simulink model "bdot_simple_sim_edits"  (R2016b)
settings: Solver=ode23tb  StartTime=0.0  StopTime=2000  RelTol=1e-3  EnableMultiTasking=on
values from neighbouring files (symbols this model uses):
  fsw_params = init_fsw_params()    [bdot_controller_edit_test.m]    (also in bdot_controlller_unit_test.m)
  sim_params = init_sim_params(fsw_params)    [bdot_controller_edit_test.m]    (also in bdot_controlller_unit_test.m)
undefined symbols (not defined in the file or in its folder): body_rates, DiscIntNeverNeededParam, Dynamics, dynamics_lib, position, quaternion, velocity
libraries: aerolibutil x11, vrlib x2, bus_stubs_template x1, environment_lib x1, bdot_controller_lib x1, magnetorquer_assembly_lib x1
settings Model: Creator=Taylor  LastModifiedBy=taylorreynolds
settings OptimizationCC: DefaultParameterBehavior=Inlined  UseDivisionForNetSlopeComputation=on  UseFloatMulNetSlope=on  InlineInvariantSignals=on  PassReuseOutputArgsAs=Individual arguments  ZeroExternalMemoryAtStartup=off  ZeroInternalMemoryAtStartup=off  NoFixptDivByZeroProtection=on  EfficientFloat2IntCast=on  LifeSpan=1
settings DebuggingCC: ParameterTunabilityLossMsg=error  SFUnexpectedBacktrackingDiag=warning  SFNoUnconditionalDefaultTransitionDiag=warning  SFExecutionAtInitializationDiag=none
settings HardwareCC: ProdBitPerInt=16  ProdBitPerPointer=16  ProdBitPerSizeT=16  ProdBitPerPtrDiffT=16  ProdLargestAtomicFloat=None  ProdWordSize=16  ProdHWDeviceType=Texas Instruments->MSP430
settings RTWCC: SystemTargetFile=ert.tlc  TemplateMakefile=ert_default_tmf  Description=Embedded Coder  GenerateReport=on  IncludeHyperlinkInReport=on  LaunchReport=on  GenerateTraceInfo=on  GenerateTraceReport=on  GenerateTraceReportSl=on  GenerateTraceReportSf=on  GenerateTraceReportEml=on  GenerateCodeMetricsReport=on
settings CodeAppCC: ForceParamTrailComments=on  IgnoreCustomStorageClasses=off  OperatorAnnotations=on  SimulinkDataObjDesc=on  SFDataObjDesc=on  MATLABFcnDesc=on  CustomSymbolStrGlobalVar=rt$N$M  CustomSymbolStrType=$N$M  CustomSymbolStrFcn=$N$M$F  CustomSymbolStrMacro=$N$M  InsertBlockDesc=on  MATLABSourceComments=on
settings ERTTargetCC: GenerateSampleERTMain=on  CombineSignalStateStructs=on  SupportComplex=off  SupportContinuousTime=on  SupportNonInlinedSFcns=on  InlinedParameterPlacement=NonHierarchical  ERTCustomFileTemplate=example_file_process.tlc  ERTFilePackagingFormat=CompactWithDataFile
settings ConfigComp: CovMetricSettings=dw  CovHtmlReporting=on  CovSaveCumulativeToWorkspaceVar=on  CovSaveSingleToWorkspaceVar=on  CovExternalEMLEnable=off

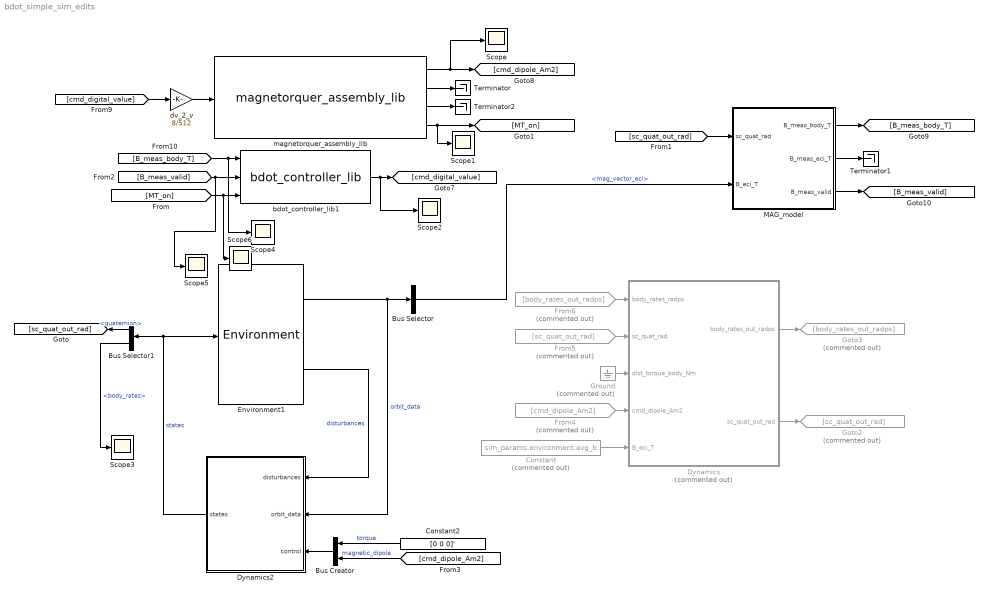
== system bdot_simple_sim_edits ==
  Bus Creator : BusCreator  Inputs=2
  Bus Selector : BusSelector  OutputSignals=mag_vector_eci
  Bus Selector1 : BusSelector  OutputSignals=quaternion,body_rates
  Constant : Constant  Commented=on  Value=sim_params.environment.avg_b
  Constant2 : Constant  Value=[0 0 0]'
  Dynamics : Subsystem  Commented=on
  Dynamics2 : Subsystem  AncestorBlock=dynamics_lib/Dynamics
  Environment1 : environment_lib/Environment
  From4 : From  Commented=on  GotoTag=cmd_dipole_Am2
  From5 : From  Commented=on  GotoTag=sc_quat_out_rad
  From6 : From  Commented=on  GotoTag=body_rates_out_radps
  Goto2 : Goto  Commented=on  GotoTag=sc_quat_out_rad
  Goto3 : Goto  Commented=on  GotoTag=body_rates_out_radps
  Ground : Ground  Commented=on
  MAG_model : Subsystem
  Scope{,1..6} (7 alike) : Scope
  Terminator : Terminator
  Terminator1 : Terminator
  Terminator2 : Terminator
  bdot_controller_lib1 : bdot_controller_lib/bdot_controller_lib
  dv_2_v : Gain  Gain=8/512
  magnetorquer_assembly_lib : magnetorquer_assembly_lib/magnetorquer_assembly_lib
  wires:
  bdot_controller_lib1/1 -> Scope2/1, [cmd_digital_value]
  [B_meas_body_T] -> Scope4/1, bdot_controller_lib1/1
  MAG_model/3(B_meas_valid) -> [B_meas_valid]
  MAG_model/1(B_meas_body_T) -> [B_meas_body_T]
  MAG_model/2(B_meas_eci_T) -> Terminator1/1
  [sc_quat_out_rad] -> MAG_model/1(sc_quat_rad)
  From6/1 -> Dynamics/1(body_rates_radps)
  Dynamics/1(body_rates_out_radps) -> Goto3/1
  Dynamics/2(sc_quat_out_rad) -> Goto2/1
  From5/1 -> Dynamics/2(sc_quat_rad)
  Ground/1 -> Dynamics/3(dist_torque_body_Nm)
  From4/1 -> Dynamics/4(cmd_dipole_Am2)
  Constant/1 -> Dynamics/5(B_eci_T)
  [B_meas_valid] -> Scope5/1, bdot_controller_lib1/2
  dv_2_v/1 -> magnetorquer_assembly_lib/1
  [cmd_digital_value] -> dv_2_v/1
  magnetorquer_assembly_lib/1 -> Scope/1, [cmd_dipole_Am2]
  magnetorquer_assembly_lib/2 -> Terminator/1
  magnetorquer_assembly_lib/4 -> Scope1/1, [MT_on]
  magnetorquer_assembly_lib/3 -> Terminator2/1
  [MT_on] -> Scope6/1, bdot_controller_lib1/3
  Environment1/1 -> Dynamics2/2(orbit_data), Bus Selector/1  "orbit_data"
  Environment1/2 -> Dynamics2/1(disturbances)  "disturbances"
  Bus Creator/1 -> Dynamics2/3(control)
  Dynamics2/1(states) -> Environment1/1, Bus Selector1/1  "states"
  Constant2/1 -> Bus Creator/1  "torque"
  [cmd_dipole_Am2] -> Bus Creator/2  "magnetic_dipole"
  Bus Selector/1 -> MAG_model/2(B_eci_T)  "<mag_vector_eci>"
  Bus Selector1/1 -> [sc_quat_out_rad]  "<quaternion>"
  Bus Selector1/2 -> Scope3/1  "<body_rates>"

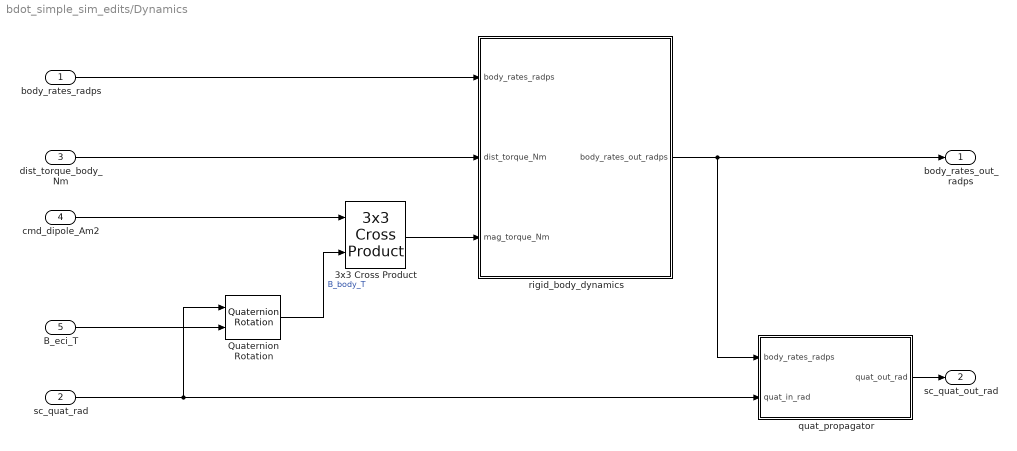
== system bdot_simple_sim_edits/Dynamics ==
  body_rates_radps : Inport
  sc_quat_rad : Inport  Port=2
  dist_torque_body_Nm : Inport  Port=3
  cmd_dipole_Am2 : Inport  Port=4
  B_eci_T : Inport  Port=5
  3x3 Cross Product : aerolibutil/3x3 Cross Product
  Quaternion Rotation : aerolibutil/Quaternion Rotation
  quat_propagator : Subsystem
  rigid_body_dynamics : Subsystem
  body_rates_out_radps : Outport
  sc_quat_out_rad : Outport  Port=2
  wires:
  Quaternion Rotation/1 -> 3x3 Cross Product/2  "B_body_T"
  cmd_dipole_Am2/1 -> 3x3 Cross Product/1
  dist_torque_body_Nm/1 -> rigid_body_dynamics/2(dist_torque_Nm)
  sc_quat_rad/1 -> Quaternion Rotation/1, quat_propagator/2(quat_in_rad)
  quat_propagator/1(quat_out_rad) -> sc_quat_out_rad/1
  body_rates_radps/1 -> rigid_body_dynamics/1(body_rates_radps)
  rigid_body_dynamics/1(body_rates_out_radps) -> body_rates_out_radps/1, quat_propagator/1(body_rates_radps)
  B_eci_T/1 -> Quaternion Rotation/2
  3x3 Cross Product/1 -> rigid_body_dynamics/3(mag_torque_Nm)

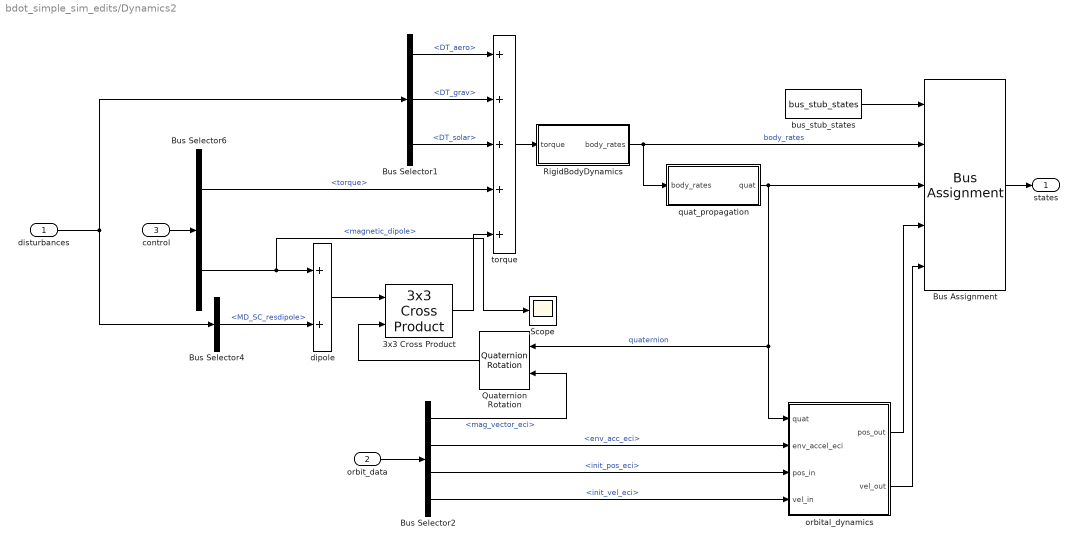
== system bdot_simple_sim_edits/Dynamics2 ==
  disturbances : Inport  OutDataTypeStr=Bus: disturbances
  orbit_data : Inport  Port=2  OutDataTypeStr=Bus: orbit_data
  control : Inport  Port=3  OutDataTypeStr=Bus: control
  3x3 Cross Product : aerolibutil/3x3 Cross Product
  Bus Assignment : BusAssignment  AssignedSignals=body_rates,quaternion,position,velocity
  Bus Selector1 : BusSelector  OutputSignals=DT_aero,DT_grav,DT_solar
  Bus Selector2 : BusSelector  OutputSignals=mag_vector_eci,env_acc_eci,init_pos_eci,init_vel_eci
  Bus Selector4 : BusSelector  OutputSignals=MD_SC_resdipole
  Bus Selector6 : BusSelector  OutputSignals=torque,magnetic_dipole
  Quaternion Rotation : aerolibutil/Quaternion Rotation
  RigidBodyDynamics : Subsystem
  Scope : Scope
  bus_stub_states : bus_stubs_template/bus_stub_states
  dipole : Sum  Inputs=2
  orbital_dynamics : Subsystem
  quat_propagation : Subsystem
  torque : Sum  Inputs=5
  states : Outport
  wires:
  orbit_data/1 -> Bus Selector2/1
  Bus Selector2/4 -> orbital_dynamics/4(vel_in)  "<init_vel_eci>"
  Bus Selector2/3 -> orbital_dynamics/3(pos_in)  "<init_pos_eci>"
  orbital_dynamics/1(pos_out) -> Bus Assignment/4
  orbital_dynamics/2(vel_out) -> Bus Assignment/5
  Bus Selector2/1 -> Quaternion Rotation/2  "<mag_vector_eci>"
  Bus Selector2/2 -> orbital_dynamics/2(env_accel_eci)  "<env_acc_eci>"
  3x3 Cross Product/1 -> torque/5
  Quaternion Rotation/1 -> 3x3 Cross Product/2
  dipole/1 -> 3x3 Cross Product/1
  torque/1 -> RigidBodyDynamics/1(torque)
  Bus Selector6/2 -> Scope/1, dipole/1  "<magnetic_dipole>"
  Bus Selector4/1 -> dipole/2  "<MD_SC_resdipole>"
  Bus Selector6/1 -> torque/4  "<torque>"
  control/1 -> Bus Selector6/1
  Bus Selector1/3 -> torque/3  "<DT_solar>"
  Bus Selector1/2 -> torque/2  "<DT_grav>"
  Bus Selector1/1 -> torque/1  "<DT_aero>"
  disturbances/1 -> Bus Selector1/1, Bus Selector4/1
  RigidBodyDynamics/1(body_rates) -> quat_propagation/1(body_rates), Bus Assignment/2  "body_rates"
  quat_propagation/1(quat) -> orbital_dynamics/1(quat), Quaternion Rotation/1, Bus Assignment/3  "quaternion"
  bus_stub_states/1 -> Bus Assignment/1
  Bus Assignment/1 -> states/1

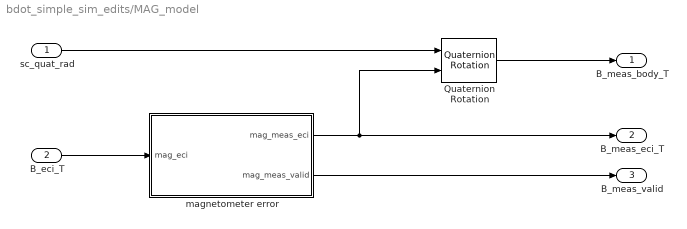
== system bdot_simple_sim_edits/MAG_model ==
  sc_quat_rad : Inport
  B_eci_T : Inport  Port=2
  Quaternion Rotation : aerolibutil/Quaternion Rotation
  magnetometer error : Subsystem
  B_meas_body_T : Outport
  B_meas_eci_T : Outport  Port=2
  B_meas_valid : Outport  Port=3
  wires:
  sc_quat_rad/1 -> Quaternion Rotation/1
  B_eci_T/1 -> magnetometer error/1(mag_eci)
  magnetometer error/1(mag_meas_eci) -> Quaternion Rotation/2, B_meas_eci_T/1
  Quaternion Rotation/1 -> B_meas_body_T/1
  magnetometer error/2(mag_meas_valid) -> B_meas_valid/1

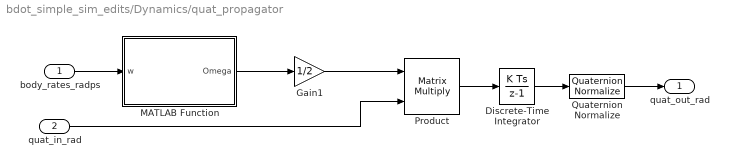
== system bdot_simple_sim_edits/Dynamics/quat_propagator ==
  body_rates_radps : Inport
  quat_in_rad : Inport  Port=2
  Discrete-Time Integrator : DiscreteIntegrator  InitialCondition=sim_params.dynamics.ic.quat_init  InitialConditionSetting=State (most efficient)  SampleTime=fsw_params.sample_time_s  ICPrevOutput=DiscIntNeverNeededParam  ICPrevScaledInput=DiscIntNeverNeededParam
  Gain1 : Gain  Gain=1/2
  MATLAB Function : MATLAB Function  TreatAsAtomicUnit=on
  Product : Product  Multiplication=Matrix(*)  RndMeth=Zero
  Quaternion Normalize : aerolibutil/Quaternion Normalize
  quat_out_rad : Outport
  wires:
  Product/1 -> Discrete-Time Integrator/1
  Quaternion Normalize/1 -> quat_out_rad/1
  Discrete-Time Integrator/1 -> Quaternion Normalize/1
  Gain1/1 -> Product/1
  quat_in_rad/1 -> Product/2
  body_rates_radps/1 -> MATLAB Function/1(w)
  MATLAB Function/1(Omega) -> Gain1/1

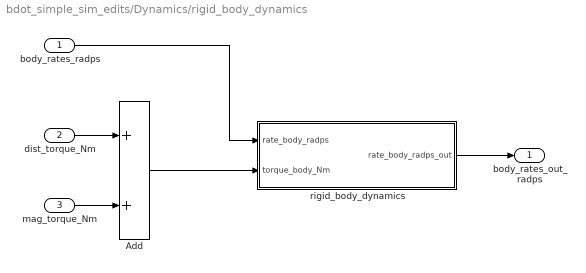
== system bdot_simple_sim_edits/Dynamics/rigid_body_dynamics ==
  body_rates_radps : Inport
  dist_torque_Nm : Inport  Port=2
  mag_torque_Nm : Inport  Port=3
  Add : Sum
  rigid_body_dynamics : Subsystem
  body_rates_out_radps : Outport
  wires:
  dist_torque_Nm/1 -> Add/1
  Add/1 -> rigid_body_dynamics/2(torque_body_Nm)
  mag_torque_Nm/1 -> Add/2
  rigid_body_dynamics/1(rate_body_radps_out) -> body_rates_out_radps/1
  body_rates_radps/1 -> rigid_body_dynamics/1(rate_body_radps)

== system bdot_simple_sim_edits/Dynamics2/RigidBodyDynamics ==
  torque : Inport
  Integrator : Integrator  InitialCondition=sim_params.dynamics.ic.rate_init
  dynamics : Subsystem
  body_rates : Outport
  wires:
  Integrator/1 -> body_rates/1, dynamics/2(omega)
  torque/1 -> dynamics/1(torque)
  dynamics/1(omega_dot) -> Integrator/1

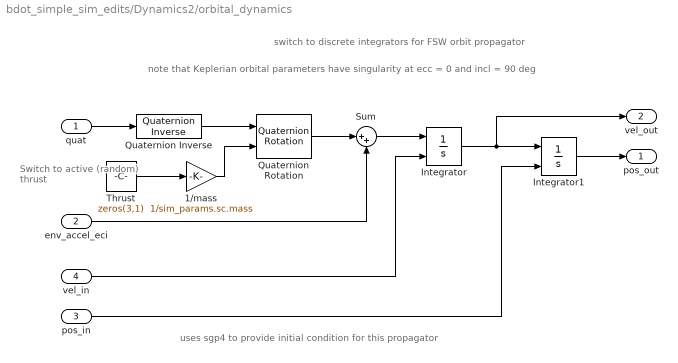
== system bdot_simple_sim_edits/Dynamics2/orbital_dynamics ==
  note: switch to discrete integrators for FSW orbit propagator
  note: note that Keplerian orbital parameters have singularity at ecc = 0 and incl = 90 deg
  note: uses sgp4 to provide initial condition for this propagator
  note: Switch to active
      | (random) thrust
  quat : Inport
  env_accel_eci : Inport  Port=2
  pos_in : Inport  Port=3
  vel_in : Inport  Port=4
  1/mass : Gain  Gain=1/sim_params.sc.mass
  Integrator : Integrator  InitialConditionSource=external  InitialCondition=sim_params.orbit.init_vel_eci
  Integrator1 : Integrator  InitialConditionSource=external  InitialCondition=sim_params.orbit.init_pos_eci
  Quaternion Inverse : aerolibutil/Quaternion Inverse
  Quaternion Rotation : aerolibutil/Quaternion Rotation
  Sum : Sum  Inputs=|++
  Thrust : Constant  Value=zeros(3,1)
  pos_out : Outport
  vel_out : Outport  Port=2
  wires:
  Integrator1/1 -> pos_out/1
  quat/1 -> Quaternion Inverse/1
  pos_in/1 -> Integrator1/2
  Quaternion Rotation/1 -> Sum/1
  Quaternion Inverse/1 -> Quaternion Rotation/1
  1/mass/1 -> Quaternion Rotation/2
  Sum/1 -> Integrator/1
  Thrust/1 -> 1/mass/1
  Integrator/1 -> Integrator1/1, vel_out/1
  env_accel_eci/1 -> Sum/2
  vel_in/1 -> Integrator/2

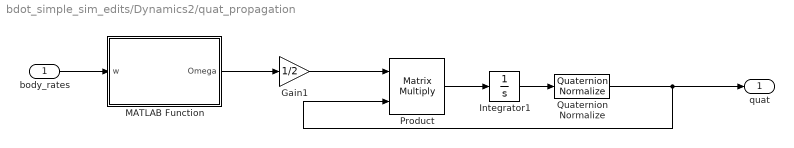
== system bdot_simple_sim_edits/Dynamics2/quat_propagation ==
  body_rates : Inport
  Gain1 : Gain  Gain=1/2
  Integrator1 : Integrator  InitialCondition=sim_params.dynamics.ic.quat_init
  MATLAB Function : MATLAB Function  TreatAsAtomicUnit=on
  Product : Product  Multiplication=Matrix(*)  RndMeth=Zero
  Quaternion Normalize : aerolibutil/Quaternion Normalize
  quat : Outport
  wires:
  Product/1 -> Integrator1/1
  Integrator1/1 -> Quaternion Normalize/1
  Gain1/1 -> Product/1
  Quaternion Normalize/1 -> quat/1, Product/2
  body_rates/1 -> MATLAB Function/1(w)
  MATLAB Function/1(Omega) -> Gain1/1

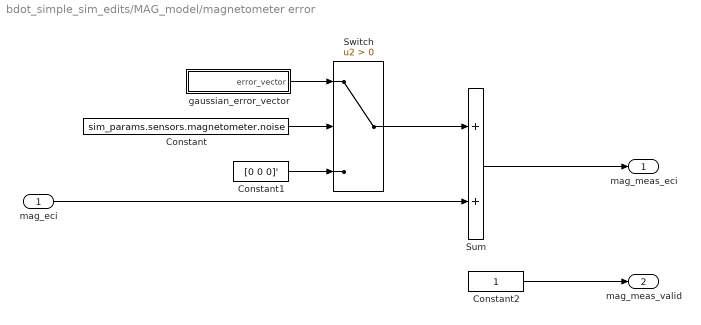
== system bdot_simple_sim_edits/MAG_model/magnetometer error ==
  mag_eci : Inport
  Constant : Constant  Value=sim_params.sensors.magnetometer.noise
  Constant1 : Constant  Value=[0 0 0]'
  Constant2 : Constant
  Sum : Sum
  Switch : Switch  Criteria=u2 > Threshold
  gaussian_error_vector : Subsystem
  mag_meas_eci : Outport
  mag_meas_valid : Outport  Port=2
  wires:
  Constant2/1 -> mag_meas_valid/1
  Switch/1 -> Sum/1
  Constant1/1 -> Switch/3
  Constant/1 -> Switch/2
  gaussian_error_vector/1(error_vector) -> Switch/1
  Sum/1 -> mag_meas_eci/1
  mag_eci/1 -> Sum/2

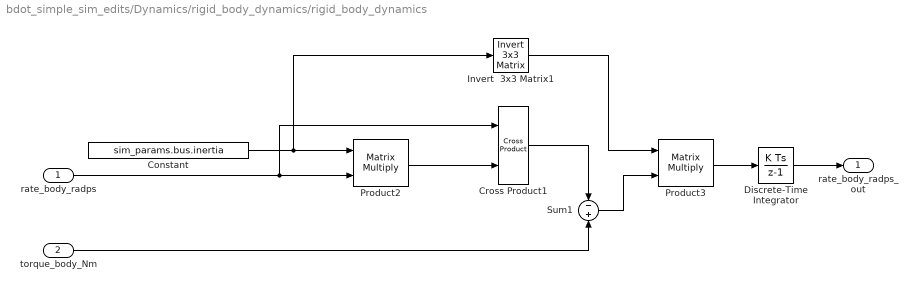
== system bdot_simple_sim_edits/Dynamics/rigid_body_dynamics/rigid_body_dynamics ==
  rate_body_radps : Inport
  torque_body_Nm : Inport  Port=2
  Constant : Constant  Value=sim_params.bus.inertia
  Cross Product1 : vrlib/Utilities/Cross Product
  Discrete-Time Integrator : DiscreteIntegrator  InitialCondition=sim_params.dynamics.ic.rate_init  InitialConditionSetting=State (most efficient)  SampleTime=fsw_params.sample_time_s  ICPrevOutput=DiscIntNeverNeededParam  ICPrevScaledInput=DiscIntNeverNeededParam
  Invert  3x3 Matrix1 : aerolibutil/Invert  3x3 Matrix
  Product2 : Product  Multiplication=Matrix(*)  RndMeth=Zero
  Product3 : Product  Multiplication=Matrix(*)  RndMeth=Zero
  Sum1 : Sum  Inputs=-+
  rate_body_radps_out : Outport
  wires:
  Discrete-Time Integrator/1 -> rate_body_radps_out/1
  Product3/1 -> Discrete-Time Integrator/1
  Invert  3x3 Matrix1/1 -> Product3/1
  Sum1/1 -> Product3/2
  torque_body_Nm/1 -> Sum1/2
  Cross Product1/1 -> Sum1/1
  rate_body_radps/1 -> Product2/2, Cross Product1/1
  Product2/1 -> Cross Product1/2
  Constant/1 -> Product2/1, Invert  3x3 Matrix1/1

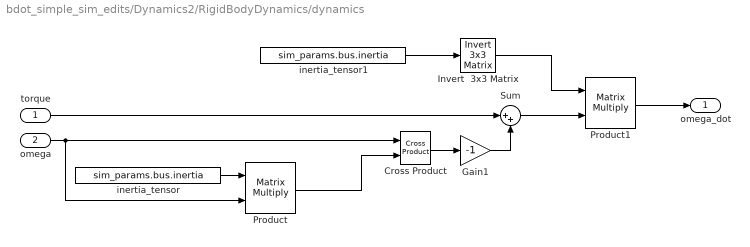
== system bdot_simple_sim_edits/Dynamics2/RigidBodyDynamics/dynamics ==
  torque : Inport
  omega : Inport  Port=2
  Cross Product : vrlib/Utilities/Cross Product
  Gain1 : Gain  Gain=-1
  Invert  3x3 Matrix : aerolibutil/Invert  3x3 Matrix
  Product : Product  Multiplication=Matrix(*)  RndMeth=Zero
  Product1 : Product  Multiplication=Matrix(*)  RndMeth=Zero
  Sum : Sum  Inputs=|++
  inertia_tensor : Constant  Value=sim_params.bus.inertia
  inertia_tensor1 : Constant  Value=sim_params.bus.inertia
  omega_dot : Outport
  wires:
  Gain1/1 -> Sum/2
  inertia_tensor1/1 -> Invert  3x3 Matrix/1
  Invert  3x3 Matrix/1 -> Product1/1
  Product1/1 -> omega_dot/1
  Sum/1 -> Product1/2
  Product/1 -> Cross Product/2
  Cross Product/1 -> Gain1/1
  inertia_tensor/1 -> Product/1
  omega/1 -> Product/2, Cross Product/1
  torque/1 -> Sum/1

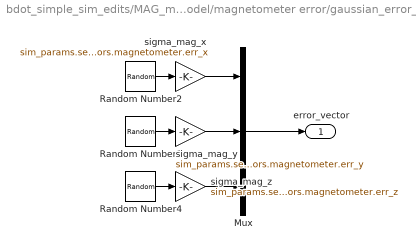
== system bdot_simple_sim_edits/MAG_model/magnetometer error/gaussian_error_vector ==
  Mux : Mux  Inputs=3
  Random Number2 : RandomNumber  SampleTime=sim_params.sensors.magnetometer.sample_time_s
  Random Number3 : RandomNumber  Seed=1  SampleTime=sim_params.sensors.magnetometer.sample_time_s
  Random Number4 : RandomNumber  Seed=2  SampleTime=sim_params.sensors.magnetometer.sample_time_s
  sigma_mag_x : Gain  Gain=sim_params.sensors.magnetometer.err_x
  sigma_mag_y : Gain  Gain=sim_params.sensors.magnetometer.err_y
  sigma_mag_z : Gain  Gain=sim_params.sensors.magnetometer.err_z
  error_vector : Outport
  wires:
  Random Number2/1 -> sigma_mag_x/1
  Random Number4/1 -> sigma_mag_z/1
  Random Number3/1 -> sigma_mag_y/1
  sigma_mag_x/1 -> Mux/1
  sigma_mag_y/1 -> Mux/2
  Mux/1 -> error_vector/1
  sigma_mag_z/1 -> Mux/3

== matlab function bdot_simple_sim_edits/Dynamics2/quat_propagation/MATLAB Function ==
  data: w input; Omega output
function Omega = skew_sym(w)
%#codegen

    w_skew = ...
        [0 w(3) -w(2);
        -w(3) 0 w(1);
        w(2) -w(1) 0];

    Omega = ...
        [0 -w';
        w w_skew];

== matlab function bdot_simple_sim_edits/Dynamics/quat_propagator/MATLAB Function ==
  data: w input; Omega output
function Omega = skew_sym(w)
%#codegen

    w_skew = ...
        [0 w(3) -w(2);
        -w(3) 0 w(1);
        w(2) -w(1) 0];

    Omega = ...
        [0 -w';
        w w_skew];
